simulink model "RLTunningTV"  (R2019b)
settings: Solver=odeN  StartTime=0.0  StopTime=15  FixedStep=0.001  RelTol=1e-3
PreLoadFcn:
  | Vehicle_parameters;
  | hcc_init;
InitFcn:
  | Vehicle_parameters;
  | hcc_init;
values from neighbouring files (symbols this model uses):
  c = (1.596+1.610)/2    (= 1.603)    [Vehicle_parameters.m]
  g = 9.8    [Vehicle_parameters.m]
  gamma = 0.006    [hcc_init.m]
  Jzz = 2050    [Vehicle_parameters.m]
  kx1 = 0.05890269    [hcc_init.m]
  ky1 = 0.04086363    [hcc_init.m]
  kz1 = 0.27516026    [hcc_init.m]
  lf = 1.3265    [Vehicle_parameters.m]
  lr = 1.3685    [Vehicle_parameters.m]
  M = 1360    [Vehicle_parameters.m]
  n = 6    [hcc_init.m]    (also in smoothing_t0.m = 16)
  pbk_gain = 1.0    (= 1)    [hcc_init.m]
  Q_gain = 50.0    (= 50)    [hcc_init.m]
  Qf = [0.0, 0.0 ... (first row only)    [hcc_init.m]
  Qr = [0.0, 0.0 ... (first row only)    [hcc_init.m]
  Reff = 0.323    [Vehicle_parameters.m]
  swa_gain = 45.0    (= 45)    [hcc_init.m]
  umax_m = 4000.0    (= 4000)    [hcc_init.m]
  umin_br = umin_m + umin_b    (= -4500)    [hcc_init.m]
  v = 80    [Vehicle_parameters.m]
  wFx = 0.4    [hcc_init.m]
  wFy = 0.02    [hcc_init.m]
  wGz = 1500.89459504    [hcc_init.m]
undefined symbols (not defined in the file or in its folder): DiscIntNeverNeededParam, LMUX, LMUY, sigbuilder_block
libraries: simulink x10, rllib x1
(part 3 of 3)

== matlab function RLTunningTV/Environment/DCIM/Tire_model/Pacejka_Fy ==
  data: Fy output; alphaFR input; alphaFL input; alphaRR input; alphaRL input; Fz_FR input; Fz_FL input; Fz_RR input; Fz_RL input
function Fy  = fcn(alphaFR , alphaFL, alphaRR, alphaRL,   Fz_FR, Fz_FL, Fz_RR, Fz_RL)

m = 1360;             % vehicle mass[kg]
g = 9.8;


%[SCALING_COEFFICIENTS]
LFZO                  	= 1;		% scale factor of nominal (rated) load
LCX                   	= 1;		% scale factor of Fx shape factor
LMUX                  	= 1;	    % scale factor of Fx peak friction coefficient
LEX                   	= 1;		% scale factor of Fx curvature factor
LKX                   	= 1;		% scale factor of Fx slip stiffness
LHX                   	= 1;	    % scale factor of Fx horizontal shfit
LVX                   	= 1;		% scale factor of Fx vertical shift
LGAX			        = 1;		% scale factor of camber for Fx  
LCY                   	= 1;		% scale factor of Fy shape factor
LMUY                  	= 1;		% scale factor of Fy peak friction coefficient
LEY                   	= 1;		% scale factor of Fy curvature factor
LKY                   	= 1;		% scale factor of Fy cornering stiffness
LHY                   	= 1;		% scale factor of Fy horizontal shift
LVY                   	= 1;		% scale factor of Fy vertical shift
LGAY                  	= 1;		% scale factor of camber for Fy
LTR                   	= 1;		% scale factor of peak of pneumatic trail
LRES                  	= 1;		% scale factor for offset of residual torque
LGAZ                  	= 1;		% scale factor of camber for Mz        
LXAL                  	= 1;		% scale factor of alpha infulence on Fx
LYKA                  	= 1;		% scale factor of kappa influence on Fy
LVYKA                 	= 1;		% scale factor of kappa induced Fy
LS                    	= 1;		% scale factor of Mz moment arm of Fx
LSGKP                 	= 1;		% scale factor of relaxation length of Fx
LSGAL                 	= 1;		% scale factor of relaxation length of Fy
LGYR                  	= 1;		% scale factor of gyroscopic torque
LMX                   	= 1;		% scale factor of overturning couple stiffness
LVMX			        = 1;		% scale factor of Mx vertical shift  
LMY                   	= 1;		% scale factor of rolling resistance torque




%[LATERAL_COEFFICIENTS]
PCY1                  	=  2.1322;	          % shape factor Cfy for lateral forces
PDY1                  	=  1.0283;	          % lateral friction Muy at FzNom
PDY2                  	= -0.16758;	          % variation of friction Muy with load
PDY3                  	= -1.5821;	          % variation of friction Muy with squared camber
PEY1                  	=  0.33443;	          % lateral curvature Efy at FzNom
PEY2                  	= -1.8733;	          % variation of curvature Efy with load
PEY3                  	= -0.13136;	          % zero order camber dependency of curvature Efy
PEY4                  	= -11.677;	          % variation of curvature Efy with camber
PKY1                  	= -20.505;	          % maximum value of stiffness Kfy/FzNom
PKY2                  	=  2.0284;	          % load at which Kfy reaches maximum value
PKY3                  	=  0.89994;	          % variation of Kfy/Fznom with camber
PHY1                  	=  0.0031377;	      % horizontal shift Shy at FzNom
PHY2                  	=  0.00051596;	      % variation of shift Shy with load
PHY3                  	=  0.039251;	      % variation of shift Shy with camber
PVY1                  	=  0.026365;	      % vertical shift in Svy/Fz at FzNom
PVY2                  	= -0.0062119;    	  % variation of shift Svy/Fz with load
PVY3                  	= -0.41389;	          % variation of shift Svy/Fz with camber
PVY4                  	= -0.048038;	      % variation of shift Svy/Fz with camber and load
RBY1                  	=  22.003;	          % slope factor for combined Fy reduction
RBY2                  	= -13.623;	          % variation of slope Fy reduction with Alpha
RBY3                  	= -0.0093616;	      % shfit term for alpha in slope Fy reduction
RCY1                  	=  0.98294;	          % shape factor for combined Fy reduction
REY1			        =  0;		          % Curvature factor of combined Fy     
REY2			        =  0;		          % Curvature factor of combined Fy with load   
RHY1                  	= -9.1492e-11;	      % shift factor for combined Fy reduction
RHY2			        =  0;		          % shift factor for combined Fy reduction with load  
RVY1                  	=  22.965;	          % kappa induced side force Svyk/Muy*Fz at FzNom
RVY2                  	=  0.37981;	          % variation of Svyk/Muy*Fz with load 
RVY3                  	=  1.8552;	          % variation of Svyk/Muy*Fz with camber
RVY4                  	=  0.08767;	          % variation of Svyk/Muy*Fz with alpha
RVY5                  	= -8.8234e-11;        % variation of Svyk/Muy*Fz with kappa
RVY6                  	=  0.90374;	          % variation of Svyk/Muy*Fz with atan(kappa)
PTY1                  	=  1.75;		      % peak value of relaxation length Sig_Alpha
PTY2                  	=  1.35;		      % shape factor for Sig_alpha

FNOMIN                	= 6500;		    % nominal wheel load


PHY1_L    = PHY1;
PHY2_L    = PHY2;
PHY1_R    = -PHY1;
PHY2_R    = -PHY2;


PVY1_L    = PVY1;
PVY2_L    = PVY2;
PVY1_R    = -PVY1;
PVY2_R    = -PVY2;

% FR

dfz_FR    =   (Fz_FR - FNOMIN)/FNOMIN ;                    
     
S_H_FR = PHY1_R + PHY2_R*dfz_FR;
alpha_y_FR = alphaFR + S_H_FR;
C_y_FR    =     PCY1 *LCY;
muy_FR    =    (PDY1 + PDY2*dfz_FR)*LMUY;
D_y_FR    =     muy_FR * Fz_FR;
% E_y_FR    =    (PEY1  + PEY2 *dfz_FR + PEY3 *dfz_FR^2)*(1 - PEY4  *sign(alpha_y_FR ))*LEY;
E_y_FR    =    (PEY1  + PEY2 *dfz_FR)*(1 - PEY3  *sign(alpha_y_FR))*LEY;
K_yk_FR   =     PKY1*FNOMIN*sin(PKY2*atan(Fz_FR/(PKY2*FNOMIN)))*LKY ;
B_y_FR    =    (K_yk_FR)/(C_y_FR*D_y_FR);

S_Vy_FR        = Fz_FR * ((PVY1_R+ PVY2_R* dfz_FR) * LVY )* LMUY ;

Fy_FR = D_y_FR*sin(C_y_FR*atan(B_y_FR*alpha_y_FR - E_y_FR*(B_y_FR*alpha_y_FR - atan(B_y_FR*alpha_y_FR))))+S_Vy_FR;

% dfz_ = 1
% FL
% Fz_FL = m*g/2;



dfz_FL    =   (Fz_FL - FNOMIN)/FNOMIN ;                    
     
S_H_FL = PHY1_L + PHY2_L*dfz_FL;
alpha_y_FL = alphaFL + S_H_FL;
C_y_FL    =     PCY1 *LCY;
muy_FL    =    (PDY1 + PDY2*dfz_FL)*LMUY;
D_y_FL    =     muy_FL * Fz_FL;
E_y_FL    =    (PEY1  + PEY2 *dfz_FL)*(1 - PEY3  *sign(alpha_y_FL))*LEY;
K_yk_FL   =     PKY1*FNOMIN*sin(PKY2*atan(Fz_FL/(PKY2*FNOMIN)))*LKY ;
B_y_FL    =    (K_yk_FL)/(C_y_FL*D_y_FL);

S_Vy_FL        = Fz_FL * ((PVY1_L+ PVY2_L* dfz_FL) * LVY )* LMUY ;


Fy_FL = D_y_FL*sin(C_y_FL*atan(B_y_FL*alpha_y_FL - E_y_FL*(B_y_FL*alpha_y_FL - atan(B_y_FL*alpha_y_FL))))+S_Vy_FL;

% RR
% Fz_RR = m*g/2;
dfz_RR    =   (Fz_RR - FNOMIN)/FNOMIN ;                    
     
S_H_RR = PHY1_R + PHY2_R*dfz_RR;
alpha_y_RR = alphaRR + S_H_RR;
C_y_RR    =     PCY1 *LCY;
muy_RR    =    (PDY1 + PDY2*dfz_RR)*LMUY;
D_y_RR    =     muy_RR * Fz_RR;
E_y_RR    =    (PEY1  + PEY2 *dfz_RR)*(1 - PEY3*sign(alpha_y_RR))*LEY;
K_yk_RR   =     PKY1*FNOMIN*sin(PKY2*atan(Fz_RR/(PKY2*FNOMIN)))*LKY ;
B_y_RR    =    (K_yk_RR)/(C_y_RR*D_y_RR);
S_Vy_RR        = Fz_RR * ((PVY1_R+ PVY2_R* dfz_RR) * LVY )* LMUY ;

Fy_RR = D_y_RR*sin(C_y_RR*atan(B_y_RR*alpha_y_RR - E_y_RR*(B_y_RR*alpha_y_RR - atan(B_y_RR*alpha_y_RR))))+S_Vy_RR;

% RL
% Fz_RL = m*g/2;
dfz_RL    =   (Fz_RL - FNOMIN)/FNOMIN ;                    
 
S_H_RL = PHY1_L + PHY2_L*dfz_RL;
alpha_y_RL = alphaRL + S_H_RL;
C_y_RL    =     PCY1 *LCY;
muy_RL    =    (PDY1 + PDY2*dfz_RL)*LMUY;
D_y_RL    =     muy_RL * Fz_RL;
E_y_RL    =    (PEY1  + PEY2 *dfz_RL)*(1 - PEY3  *sign(alpha_y_RL))*LEY;
K_yk_RL   =     PKY1*FNOMIN*sin(PKY2*atan(Fz_RL/(PKY2*FNOMIN)))*LKY ;
B_y_RL    =    (K_yk_RL)/(C_y_RL*D_y_RL);
S_Vy_RL        = Fz_RL * ((PVY1_L+ PVY2_L* dfz_RL) * LVY )* LMUY ;

Fy_RL = D_y_RL*sin(C_y_RL*atan(B_y_RL*alpha_y_RL - E_y_RL*(B_y_RL*alpha_y_RL - atan(B_y_RL*alpha_y_RL))))+S_Vy_RL;

Fy = [Fy_FR, Fy_FL, Fy_RR, Fy_RL]';
muy = [muy_FR, muy_FL, muy_RR, muy_RL]';

== matlab function RLTunningTV/Environment/MATLAB Function ==
  data: Fz input; Fx input; Fy input; mu input; maxQ input; minQ input; road_wheel input; ERR input; weights input; wxd_weights input; gains input; Q_gain input; P1 output
function P1   = fcn(Fz, Fx, Fy, mu, maxQ, minQ,...
                 road_wheel, ERR, weights,...
                 wxd_weights, gains, Q_gain)

d_Q = zeros(4,1);             
P1 = zeros(1,1);             
Fz1 = Fz(1);
Fz2 = Fz(2);
Fz3 = Fz(3);
Fz4 = Fz(4);

Fx1 = Fx(1);
Fx2 = Fx(2);
Fx3 = Fx(3);
Fx4 = Fx(4);

Fy1 = Fy(1);
Fy2 = Fy(2);
Fy3 = Fy(3);
Fy4 = Fy(4);

mux1 = mu(1);
mux2 = mu(2);
mux3 = mu(3);
mux4 = mu(4);
muy1 = mu(5);
muy2 = mu(6);
muy3 = mu(7);
muy4 = mu(8);

Q1_max = maxQ(1);
Q2_max = maxQ(2);
Q3_max = maxQ(3);
Q4_max = maxQ(4);

Q1_min = minQ(1);
Q2_min = minQ(2);
Q3_min = minQ(3);
Q4_min = minQ(4);

delta_FR = road_wheel(1);
delta_FL = road_wheel(2);
delta_RR = 0;
delta_RL = 0;

Ex = ERR(1);
Ey = ERR(2);
Ez = ERR(3);

wFx = weights(1);
wFy = weights(2);
wGz = weights(3);

wxd1 = wxd_weights(1);
wxd2 = wxd_weights(2);
wxd3 = wxd_weights(3);
wxd4 = wxd_weights(4);

gamma  = gains(1);
n      = gains(2);

Qgain = Q_gain;


Fx_max1  =mux1*Fz1;
Fy_max1  =muy1*Fz1;
Fx_max2  =mux2*Fz2;
Fy_max2  =muy2*Fz2;
Fx_max3  =mux3*Fz3;
Fy_max3  =muy3*Fz3;
Fx_max4  =mux4*Fz4;
Fy_max4  =muy4*Fz4;

ro21 = ((Fx1/Fx_max1)^2+(Fy1/Fy_max1)^2);
ro22 = ((Fx2/Fx_max2)^2+(Fy2/Fy_max2)^2);
ro23 = ((Fx3/Fx_max3)^2+(Fy3/Fy_max3)^2);
ro24 = ((Fx4/Fx_max4)^2+(Fy4/Fy_max4)^2);
    
    
wf1=gamma*(ro21^n); 
wf2=gamma*(ro22^n);
wf3=gamma*(ro23^n);
wf4=gamma*(ro24^n);
   
lf = 1.509;
lr = 1.231;
c = 1.32;
g = 9.8;
Reff = 0.3;
  

if (Fx1 > 0)
			wf1 = wf1 + gamma*((Reff*Fx1/Q1_max)^2*n);
	else    wf1 = wf1 + gamma*((Reff*Fx1/Q1_min)^2*n);
end 
if (Fx2 > 0)
			wf2 = wf2 + gamma*((Reff*Fx2/Q2_max)^2*n);
	else    wf2 = wf2 + gamma*((Reff*Fx2/Q2_min)^2*n);
end   
if (Fx3 > 0)
			wf3 = wf3 + gamma*((Reff*Fx3/Q3_max)^2*n);
	else    wf3 = wf3 + gamma*((Reff*Fx3/Q3_min)^2*n);
end  
if (Fx4 > 0)
			wf4 = wf4 + gamma*((Reff*Fx4/Q4_max)^2*n);
	else    wf4 = wf4 + gamma*((Reff*Fx4/Q4_min)^2*n);
end            
             
Jac = [cos(delta_FL), cos(delta_FR), 1, 1;...
       sin(delta_FL), sin(delta_FR), 0, 0;...
       lf*sin(delta_FL)-c*cos(delta_FL), lf*sin(delta_FR)+c*cos(delta_FR), -c, c];
   
   
E = [Ex, Ey, Ez]';
      
F = [Fx1, Fx2, Fx3, Fx4]';

WE = [wFx, 0, 0;...
      0, wFy, 0;...
      0,  0, wGz];
  
Wdf = [wxd1,0 ,0 ,0;...
       0 , wxd2,0 ,0;...
       0, 0, wxd3, 0;...
       0, 0, 0, wxd4];  
   

Wf = [wf1, 0, 0, 0;...
      0, wf2, 0, 0;...
      0, 0, wf3, 0;...
      0, 0,  0, wf4];

  
den = Wf + Wdf + (Jac'*WE)*Jac;
num = (Jac'*WE)*E - Wf*F;

df = den\num;

P1 = 1/2*((E - Jac*df)'*WE*(E - Jac*df) + df'*Wdf*df + (F+df)'*Wf*(F+df));


dQ = zeros(4,1);

dQ(1,:) = df(1,:)*Reff*Qgain;
dQ(2,:) = df(2,:)*Reff*Qgain;
dQ(3,:) = df(3,:)*Reff*Qgain;
dQ(4,:) = df(4,:)*Reff*Qgain;

d_Q = [dQ(1,:), dQ(2,:), dQ(3,:), dQ(4,:)]';
